simulink model "assignment3"  (R2020b)
settings: Solver=VariableStepAuto  StartTime=0.0  StopTime=25  RelTol=1e-3
InitFcn:
  | g = 32.18;
  | v0 = 88;
  | Rr = 15/12;
  | Kf = 1;
  | m = 50;
  | PBmax = 1500;
  | TB = 0.01;
  | I = 5;
  | slip = (0:.05:1.0);
  | mu = [0 .4 .8 .97 1.0 .98 .96 .94 .92 .9 .88 .855 .83 .81 .79 .77 .75 .73 .72 .71 .7];
  | ctrl = 1;
undefined symbols (not defined in the file): sigbuilder_block
settings Model: Creator=Sudhanshu  LastModifiedBy=Sudhanshu

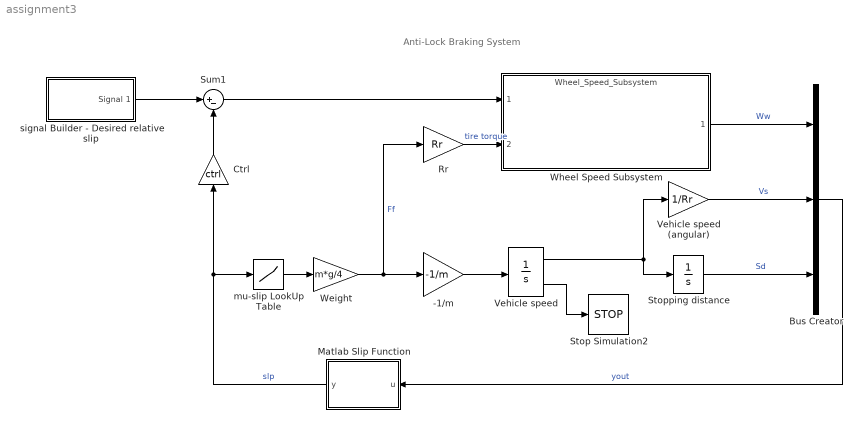
== system assignment3 ==
  note: Anti-Lock Braking System
  -1/m : Gain  Gain=-1/m  SaturateOnIntegerOverflow=on  OutDataTypeStr=Inherit: Same as input  ParamDataTypeStr=Inherit: Same as input
  Bus Creator : BusCreator  Inputs=3
  Ctrl : Gain  Gain=ctrl  SaturateOnIntegerOverflow=on  OutDataTypeStr=Inherit: Same as input  ParamDataTypeStr=Inherit: Same as input
  Matlab Slip Function : MATLAB Function  TreatAsAtomicUnit=on
  Rr : Gain  Gain=Rr  SaturateOnIntegerOverflow=on  OutDataTypeStr=Inherit: Same as input  ParamDataTypeStr=Inherit: Same as input
  Stop Simulation2 : Stop
  Stopping distance : Integrator  UpperSaturationLimit=1000  LowerSaturationLimit=0
  Sum1 : Sum  Inputs=|+-  InputSameDT=on  SaturateOnIntegerOverflow=on  OutDataTypeStr=Inherit: Same as first input
  Vehicle speed : Integrator  InitialCondition=v0  LimitOutput=on  UpperSaturationLimit=1000  LowerSaturationLimit=0  ShowSaturationPort=on
  Vehicle speed (angular) : Gain  Gain=1/Rr  SaturateOnIntegerOverflow=on  OutDataTypeStr=Inherit: Same as input  ParamDataTypeStr=Inherit: Same as input
  Weight : Gain  Gain=m*g/4  SaturateOnIntegerOverflow=on  OutDataTypeStr=Inherit: Same as input  ParamDataTypeStr=Inherit: Same as input
  Wheel Speed Subsystem : ModelReference  ModelNameDialog=Wheel_Speed_Subsystem  SimulationMode=Normal  ModelReferenceVersion=1.8
  mu-slip LookUp Table : Lookup_n-D  NumberOfTableDimensions=1  BreakpointsForDimension1=[0:.05:1.0]  Table=[0 .4 .8 .97 1.0 .98 .96 .94 .92 .9 .88 .855 .83 .81 .79 .77 .75 .73 .72 .71 .7]  SaturateOnIntegerOverflow=on  InputSameDT=on
  signal Builder - Desired relative slip : Subsystem  Tag=STV Subsys  LoadFcn=sigbuilder_block('load');  StartFcn=sigbuilder_block('start');  StopFcn=sigbuilder_block('stop');  ClipboardFcn=sigbuilder_block('clipboard');  mask(Sigbuilder block){tuvar=[0:10]}
      mask help: Simulink:masks:SigbuilderBlock_MD
      mask init:
      | if ~strcmp(get_param(bdroot(gcbh),'SimulationStatus'),'stopped') tuvar = sigbuilder_block('maskInit'); end
      settings: CopyFcn=sigbuilder_block('copy');  DeleteFcn=sigbuilder_block('delete');  ModelCloseFcn=sigbuilder_block('modelClose');  PreSaveFcn=sigbuilder_block('preSave');  PauseFcn=sigbuilder_block('pause');  ContinueFcn=sigbuilder_block('continue');  NameChangeFcn=sigbuilder_block('namechange');  OpenFcn=sigbuilder_block('open',[387 76.5 544.5 355.5 ]);  CloseFcn=sigbuilder_block('close');
      mask Display: plot(0, 0, 100, 100,[2, 2, 32, 32, 2], [68, 8, 8, 68, 68],[32, 2], [38, 38], [32, 19, 2],[53, 60, 44], [32, 17, 17, 2],[16, 16, 31, 31]);txt = getActiveGroup(gcbh);text(2, 100, txt,'verticalAlignment', 'top');
  wires:
  Stopping distance/1 -> Bus Creator/3  "Sd"
  Vehicle speed (angular)/1 -> Bus Creator/2  "Vs"
  Bus Creator/1 -> Matlab Slip Function/1(u)  "yout"
  -1/m/1 -> Vehicle speed/1
  Vehicle speed/2 -> Stop Simulation2/1
  mu-slip LookUp Table/1 -> Weight/1
  Vehicle speed/1 -> Vehicle speed (angular)/1, Stopping distance/1
  Rr/1 -> Wheel Speed Subsystem/2  "tire torque"
  Matlab Slip Function/1(y) -> Ctrl/1, mu-slip LookUp Table/1  "slp"
  Ctrl/1 -> Sum1/2
  Weight/1 -> Rr/1, -1/m/1  "Ff"
  Sum1/1 -> Wheel Speed Subsystem/1
  Wheel Speed Subsystem/1 -> Bus Creator/1  "Ww"
  signal Builder - Desired relative slip/1(Signal 1) -> Sum1/1

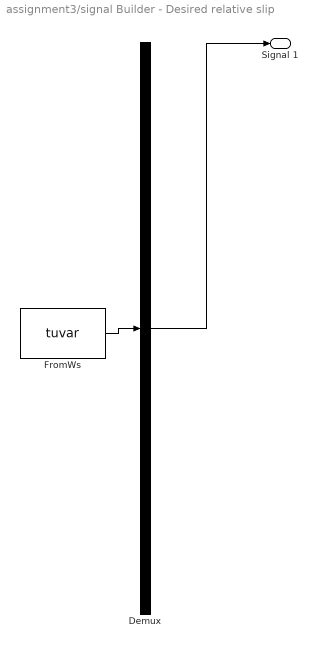
== system assignment3/signal Builder - Desired relative slip ==
  Demux : Demux  Tag=STV Demux  Outputs=1
      settings: DisplayOption=none
  FromWs : FromWorkspace  Tag=STV FromWs  VariableName=tuvar
      SigBuilderData=|
      | common.afterFinalStr = 'Extrapolate'
      | common.sampleTime = 0
      | dataSet.timeRange = [0 25]
      | dataSet.name = 'Group 1'
      | sbobj.Groups.Name = 'Group 1'
      | sbobj.Groups.Signals.Name = 'Signal 1'
      | sbobj.Groups.Signals.XData = [0 5 10 15 20 25]
      | sbobj.Groups.Signals.YData = [0.1 0.1005 0.2 0.2 0.3 0.3]
      | sbobj.Groups.TimeRange = [0 25]
  Signal 1 : Outport  Tag=STV Outport
  wires:
  Demux/1 -> Signal 1/1
  FromWs/1 -> Demux/1

== matlab function assignment3/Matlab Slip Function ==
  data: u input; y output
function y = relativeslip(u)
u = 1.0 - u(1)/(u(2) + (u(2)==0)*eps);
y = u;
